simulink model "proj2b"  (R2014a)
settings: Solver=FixedStepDiscrete  StartTime=0.0  StopTime=10.0  FixedStep=1  RelTol=1e-3
libraries: hdlsllib x6
settings Model: Creator=sahara.m  LastModifiedBy=sahara.m
settings OptimizationCC: BlockReduction=off  ConditionallyExecuteInputs=off  InlineParams=on
settings DebuggingCC: AlgebraicLoopMsg=error
settings HardwareCC: ProdHWDeviceType=ASIC/FPGA->ASIC/FPGA  ProdEqTarget=off

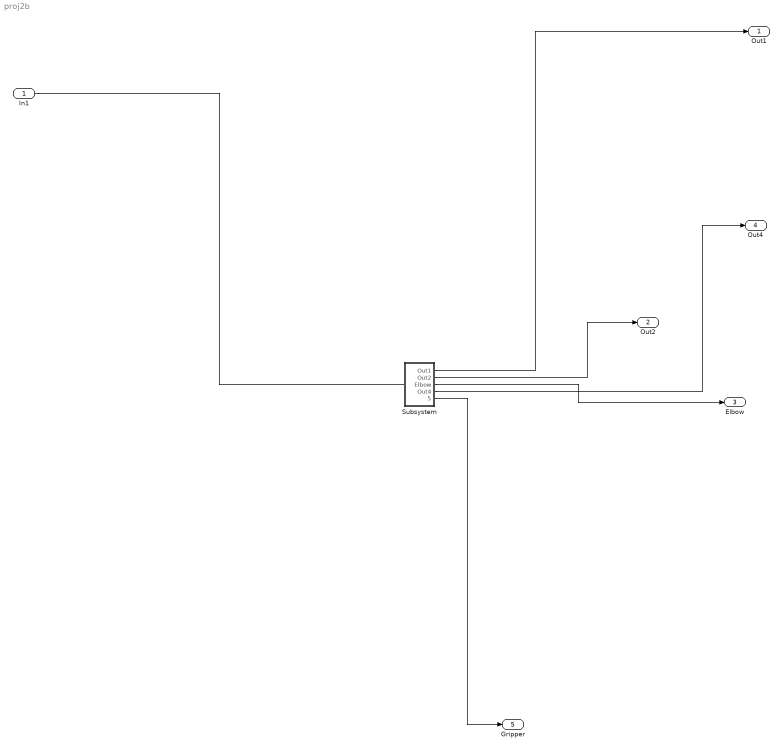
== system proj2b ==
  In1 : Inport  SampleTime=1
  Subsystem : Subsystem  TreatAsAtomicUnit=on
  Out1 : Outport  OutDataTypeStr=boolean  SampleTime=1
  Out2 : Outport  Port=2  OutDataTypeStr=boolean  SampleTime=1
  Elbow : Outport  Port=3  OutDataTypeStr=boolean  SampleTime=1
  Out4 : Outport  Port=4  OutDataTypeStr=boolean  SampleTime=1
  Gripper : Outport  Port=5  OutDataTypeStr=boolean  SampleTime=1
  wires:
  In1/1 -> ?
  Subsystem/1(Out1) -> Out1/1
  Subsystem/2(Out2) -> Out2/1
  Subsystem/3(Elbow) -> Elbow/1
  Subsystem/4(Out4) -> Out4/1
  Subsystem/5(Gripper) -> Gripper/1

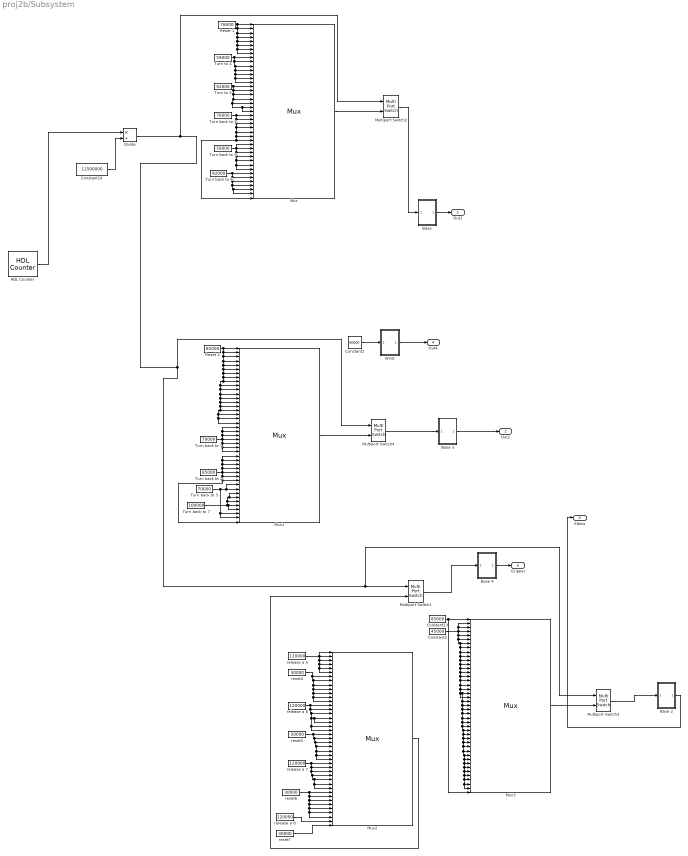
== system proj2b/Subsystem ==
  "Base " : Subsystem
  Base 2 : Subsystem
  Base 3 : Subsystem
  Base 4 : Subsystem
  Constant1 : Constant  Value=80000  OutDataTypeStr=uint32
  Constant10 : Constant  Value=12500000  VectorParams1D=off  OutDataTypeStr=uint32
  Constant13 : Constant  Value=85000  VectorParams1D=off  OutDataTypeStr=uint32
  Constant2 : Constant  Value=45000  VectorParams1D=off  OutDataTypeStr=uint32
  Divide : Product  Inputs=*/  OutDataTypeStr=uint32  RndMeth=Simplest  SaturateOnIntegerOverflow=on
  HDL Counter : hdlsllib/HDL Operations/HDL Counter  CountType=Count limited  CountInit=0  CountStep=1  CountMax=600000000  CountFromType=Initial value  CountFrom=0  CountResetPort=off  CountLoadPort=off  CountEnbPort=off  CountDirPort=off  CountDataType=Unsigned  CountWordLen=32  CountFracLen=0  CountSampTime=1
  Multiport Switch{1..4} (4 alike) : MultiPortSwitch  DataPortOrder=Zero-based contiguous  Inputs=1
  Mux{,1..3} (4 alike) : Mux  Inputs=43
  Reset 1 : Constant  Value=76000  OutDataTypeStr=uint32
  Reset 2 : Constant  Value=85000  OutDataTypeStr=uint32
  Turn back to 1 : Constant  Value=70000  OutDataTypeStr=uint32
  Turn back to 2 : Constant  Value=85000  OutDataTypeStr=uint32
  Turn back to 3 : Constant  Value=70000  OutDataTypeStr=uint32
  Turn back to 4 : Constant  Value=76000  OutDataTypeStr=uint32
  Turn back to 5 : Constant  Value=59000  OutDataTypeStr=uint32
  Turn back to 6 : Constant  Value=92000  OutDataTypeStr=uint32
  Turn back to 7 : Constant  Value=100000  OutDataTypeStr=uint32
  Turn to 4 : Constant  Value=59000  OutDataTypeStr=uint32
  Turn to 5 : Constant  Value=92000  OutDataTypeStr=uint32
  Wrist : Subsystem
  release a {5..8} (4 alike) : Constant  Value=120000  OutDataTypeStr=uint32
  reset{4..7} (4 alike) : Constant  Value=30000  OutDataTypeStr=uint32
  Out1 : Outport  OutDataTypeStr=boolean  SampleTime=1
  Out2 : Outport  Port=2  OutDataTypeStr=boolean  SampleTime=1
  Elbow : Outport  Port=3  OutDataTypeStr=boolean  SampleTime=1
  Out4 : Outport  Port=4  OutDataTypeStr=boolean  SampleTime=1
  Gripper : Outport  Port=5  OutDataTypeStr=boolean  SampleTime=1
  wires:
  "Base "/1(Out1) -> Out1/1
  Base 3/1(Out1) -> Out2/1
  Base 4/1(Out1) -> Gripper/1
  Base 2/1(Out1) -> Elbow/1
  Constant1/1 -> Wrist/1(In1)
  Wrist/1(Out1) -> Out4/1
  Multiport Switch4/1 -> Base 3/1(In1)
  Constant10/1 -> Divide/2
  HDL Counter/1 -> Divide/1
  Divide/1 -> Multiport Switch2/1, Multiport Switch3/1, Multiport Switch1/1, Multiport Switch4/1
  Reset 1/1 -> Mux/1, Mux/2, Mux/3, Mux/4, Mux/5, Mux/6, Mux/7, Mux/8
  Turn to 4/1 -> Mux/15, Mux/14, Mux/13, Mux/12, Mux/11, Mux/10, Mux/9
  Turn to 5/1 -> Mux/18, Mux/19, Mux/22, Mux/21, Mux/20, Mux/17, Mux/16
  Turn back to 4/1 -> Mux/29, Mux/43, Mux/28, Mux/27, Mux/26, Mux/25, Mux/24, Mux/23
  Turn back to 5/1 -> Mux/30, Mux/36, Mux/35, Mux/34, Mux/33, Mux/32, Mux/31
  Turn back to 6/1 -> Mux/42, Mux/41, Mux/40, Mux/39, Mux/38, Mux/37
  Mux/1 -> Multiport Switch2/2
  Multiport Switch2/1 -> "Base "/1(In1)
  Reset 2/1 -> Mux1/1, Mux1/2, Mux1/3, Mux1/4, Mux1/5, Mux1/6, Mux1/18, Mux1/19, Mux1/17, Mux1/16, Mux1/15, Mux1/14, Mux1/13, Mux1/12, Mux1/11, Mux1/10, Mux1/9, Mux1/8, Mux1/7
  Turn back to 1/1 -> Mux1/26, Mux1/25, Mux1/24, Mux1/23, Mux1/20, Mux1/21, Mux1/22
  Turn back to 2/1 -> Mux1/27, Mux1/28, Mux1/29, Mux1/30, Mux1/43, Mux1/33, Mux1/32, Mux1/31
  Mux1/1 -> Multiport Switch4/2
  Turn back to 3/1 -> Mux1/41, Mux1/42, Mux1/34, Mux1/35
  Turn back to 7/1 -> Mux1/40, Mux1/39, Mux1/38, Mux1/36, Mux1/37
  release a 5/1 -> Mux2/6, Mux2/5, Mux2/4, Mux2/3, Mux2/2, Mux2/1
  reset4/1 -> Mux2/13, Mux2/12, Mux2/11, Mux2/10, Mux2/9, Mux2/8, Mux2/7
  release a 6/1 -> Mux2/20, Mux2/19, Mux2/18, Mux2/17, Mux2/16, Mux2/15, Mux2/14
  reset5/1 -> Mux2/27, Mux2/26, Mux2/25, Mux2/24, Mux2/23, Mux2/22, Mux2/21
  release a 7/1 -> Mux2/34, Mux2/33, Mux2/32, Mux2/31, Mux2/30, Mux2/29, Mux2/28
  reset6/1 -> Mux2/41, Mux2/40, Mux2/39, Mux2/38, Mux2/37, Mux2/36, Mux2/35
  release a 8/1 -> Mux2/42
  reset7/1 -> Mux2/43
  Mux2/1 -> Multiport Switch1/2
  Multiport Switch1/1 -> Base 4/1(In1)
  Mux3/1 -> Multiport Switch3/2
  Multiport Switch3/1 -> Base 2/1(In1)
  Constant13/1 -> Mux3/43, Mux3/1
  Constant2/1 -> Mux3/18, Mux3/20, Mux3/42, Mux3/41, Mux3/40, Mux3/39, Mux3/38, Mux3/37, Mux3/36, Mux3/35, Mux3/34, Mux3/33, Mux3/32, Mux3/31, Mux3/30, Mux3/29, Mux3/28, Mux3/27, Mux3/26, Mux3/25, Mux3/24, Mux3/23, Mux3/22, Mux3/21, Mux3/19, Mux3/17, Mux3/16, Mux3/15, Mux3/14, Mux3/13, Mux3/12, Mux3/11, Mux3/10, Mux3/9, Mux3/8, Mux3/7, Mux3/6, Mux3/5, Mux3/4, Mux3/3, Mux3/2

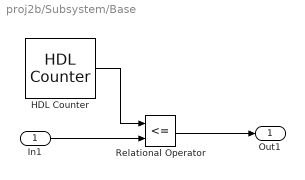
== system proj2b/Subsystem/Base  ==
  In1 : Inport  OutDataTypeStr=uint32  SampleTime=1
  HDL Counter : hdlsllib/HDL Operations/HDL Counter  CountType=Count limited  CountInit=0  CountStep=1  CountMax=1000000  CountFromType=Initial value  CountFrom=0  CountResetPort=off  CountLoadPort=off  CountEnbPort=off  CountDirPort=off  CountDataType=Unsigned  CountWordLen=24  CountFracLen=0  CountSampTime=1
  Relational Operator : RelationalOperator  Operator=<=  OutDataTypeStr=boolean
  Out1 : Outport  OutDataTypeStr=boolean  SampleTime=1
  wires:
  Relational Operator/1 -> Out1/1
  HDL Counter/1 -> Relational Operator/1
  In1/1 -> Relational Operator/2

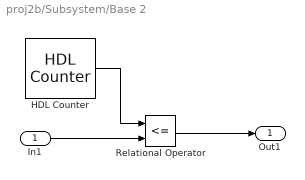
== system proj2b/Subsystem/Base 2 ==
  In1 : Inport  OutDataTypeStr=uint32  SampleTime=1
  HDL Counter : hdlsllib/HDL Operations/HDL Counter  CountType=Count limited  CountInit=0  CountStep=1  CountMax=1000000  CountFromType=Initial value  CountFrom=0  CountResetPort=off  CountLoadPort=off  CountEnbPort=off  CountDirPort=off  CountDataType=Unsigned  CountWordLen=24  CountFracLen=0  CountSampTime=1
  Relational Operator : RelationalOperator  Operator=<=  OutDataTypeStr=boolean
  Out1 : Outport  OutDataTypeStr=boolean  SampleTime=1
  wires:
  Relational Operator/1 -> Out1/1
  HDL Counter/1 -> Relational Operator/1
  In1/1 -> Relational Operator/2

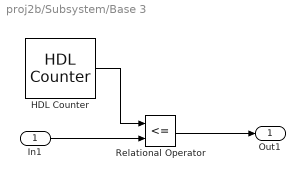
== system proj2b/Subsystem/Base 3 ==
  In1 : Inport  OutDataTypeStr=uint32  SampleTime=1
  HDL Counter : hdlsllib/HDL Operations/HDL Counter  CountType=Count limited  CountInit=0  CountStep=1  CountMax=1000000  CountFromType=Initial value  CountFrom=0  CountResetPort=off  CountLoadPort=off  CountEnbPort=off  CountDirPort=off  CountDataType=Unsigned  CountWordLen=24  CountFracLen=0  CountSampTime=1
  Relational Operator : RelationalOperator  Operator=<=  OutDataTypeStr=boolean
  Out1 : Outport  OutDataTypeStr=boolean  SampleTime=1
  wires:
  Relational Operator/1 -> Out1/1
  HDL Counter/1 -> Relational Operator/1
  In1/1 -> Relational Operator/2

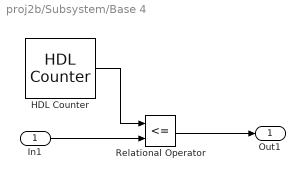
== system proj2b/Subsystem/Base 4 ==
  In1 : Inport  OutDataTypeStr=uint32  SampleTime=1
  HDL Counter : hdlsllib/HDL Operations/HDL Counter  CountType=Count limited  CountInit=0  CountStep=1  CountMax=1000000  CountFromType=Initial value  CountFrom=0  CountResetPort=off  CountLoadPort=off  CountEnbPort=off  CountDirPort=off  CountDataType=Unsigned  CountWordLen=24  CountFracLen=0  CountSampTime=1
  Relational Operator : RelationalOperator  Operator=<=  OutDataTypeStr=boolean
  Out1 : Outport  OutDataTypeStr=boolean  SampleTime=1
  wires:
  Relational Operator/1 -> Out1/1
  HDL Counter/1 -> Relational Operator/1
  In1/1 -> Relational Operator/2

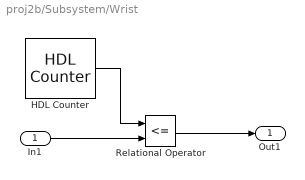
== system proj2b/Subsystem/Wrist ==
  In1 : Inport  OutDataTypeStr=uint32  SampleTime=1
  HDL Counter : hdlsllib/HDL Operations/HDL Counter  CountType=Count limited  CountInit=0  CountStep=1  CountMax=1000000  CountFromType=Initial value  CountFrom=0  CountResetPort=off  CountLoadPort=off  CountEnbPort=off  CountDirPort=off  CountDataType=Unsigned  CountWordLen=24  CountFracLen=0  CountSampTime=1
  Relational Operator : RelationalOperator  Operator=<=  OutDataTypeStr=boolean
  Out1 : Outport  OutDataTypeStr=boolean  SampleTime=1
  wires:
  Relational Operator/1 -> Out1/1
  HDL Counter/1 -> Relational Operator/1
  In1/1 -> Relational Operator/2
